simulink model "verify_Hot_Water_T_Mdot_Profile_mdl"  (R2018b)
settings: Solver=ode45  StartTime=0.0  StopTime=24*3600  MaxStep=900  RelTol=1e-3  EnableMultiTasking=on
undefined symbols (not defined in the file or in its folder): path_carnot
libraries: carnot x5
settings Model: DEBUGGLOBALLEVEL=DEBUGLEVEL  DEBUGMAXTOTALWARNINGS=0  DEBUGMAXCONSECUTIVEWARNINGS=0  DEBUGWRITETOFILE=0  DEBUGFILENAME='error.txt'  Creator=drhf  LastModifiedBy=P41573
settings DataIOCC: SaveFormat=Array  SignalLoggingSaveFormat=ModelDataLogs
settings OptimizationCC: ExpressionDepthLimit=2147483647  LifeSpan=inf
settings DebuggingCC: UnderspecifiedInitializationDetection=Classic  MergeDetectMultiDrivingBlocksExec=none  SolverPrmCheckMsg=warning  FcnCallInpInsideContextMsg=warning  StateNameClashWarn=warning  SFUnexpectedBacktrackingDiag=warning  SFNoUnconditionalDefaultTransitionDiag=warning  SFExecutionAtInitializationDiag=none
settings HardwareCC: ProdBitPerPointer=32  ProdBitPerSizeT=32  ProdBitPerPtrDiffT=32  ProdLargestAtomicFloat=None  ProdIntDivRoundTo=Undefined  ProdEndianess=Unspecified  ProdWordSize=32  ProdHWDeviceType=32-bit Generic
settings ModelReferenceCC: PropagateSignalLabelsOutOfModel=off
settings SFSimCC: SimUseLocalCustomCode=off
settings RTWCC: RTWUseLocalCustomCode=off
settings CodeAppCC: StateflowObjectComments=on
settings GRTTargetCC: TargetLangStandard=C89/C90 (ANSI)  GeneratePreprocessorConditionals=Disable all  CombineOutputUpdateFcns=off  GRTInterface=on
settings ConfigComp: CovMetricSettings=dw  CovHtmlReporting=on  CovSaveCumulativeToWorkspaceVar=on  CovSaveSingleToWorkspaceVar=on  CovExternalEMLEnable=off

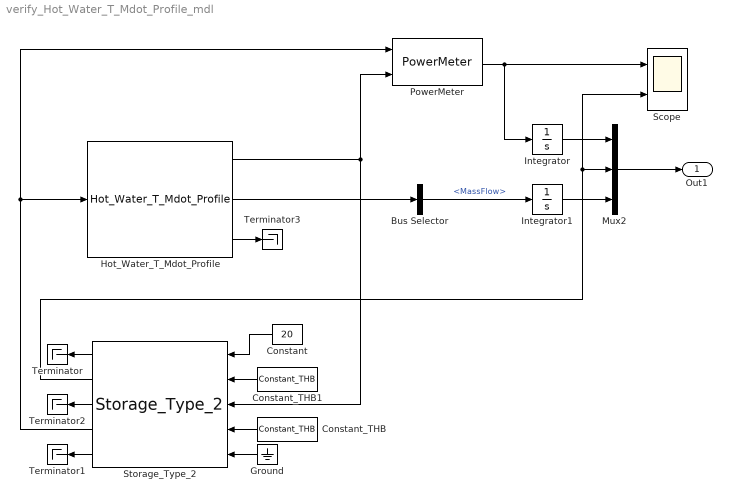
== system verify_Hot_Water_T_Mdot_Profile_mdl ==
  Bus Selector : BusSelector  OutputSignals=MassFlow
  Constant : Constant  Value=20
  Constant_THB : carnot/Source/Simple/Constant_THB  t=40  mdot=0*100/3600  p=1e5  mID=No Pressure Drop  fluid=Water  mix=0  mix2=0  mix3=0  dia=0.02  hgt=0
      settings: SourceProductName=Carnot
  Constant_THB1 : carnot/Source/Simple/Constant_THB  t=60  mdot=1000/3600  p=1e5  mID=No Pressure Drop  fluid=Water  mix=0  mix2=0  mix3=0  dia=0.02  hgt=0
      settings: SourceProductName=Carnot
  Ground : Ground
  Hot_Water_T_Mdot_Profile : carnot/Load/Hot_Water_Tapping/Hot_Water_T_Mdot_Profile  VariantControl=Variant3  Thot=45  Tcold=10  Tamp=0  dshift=-137  period="24*3600   % one day"  rep_seq_t="[7 12 19]*3600  % tapping at 7:00, 12:00 and 19:00"  rep_seq_d="[0.2 0.1 0.2]*3600  % total duration is 1/2 h"  rep_seq_y="[1 1 1]*200/1800   % 200 kg in 1/2 h"
      settings: SourceProductName=Carnot
  Integrator : Integrator
  Integrator1 : Integrator
  Mux2 : Mux  Inputs=3
  PowerMeter : carnot/Control/PowerMeter
      settings: SourceProductName=Carnot
  Scope : Scope  NumInputPorts=2
  Storage_Type_2 : carnot/Storage/Thermal/Storage_Type_2  t0=60  hgt=1.5279  stgtype=2  tini=[60 60 60 60 60 60 60 60 60 60]  mpts=[1 2 3 4 5 6 7 8 9 10]  PathName=fullfile(path_carnot('libsl'),'Storage','Thermal','Storage_Type_2','parameter_set')  FileName='StorageType2_300_L.mat'  userPath=off  userParam=off  uwall=1  ubot=1  utop=1  axcond=1  volume=0.3  dia=0.5  standing=standing cylinder  nodes=10  mpoints=10  Tsensor=0.5  hx1inlet=0.45  hx1outlet=0  hx1dia=0.03  hx1uac=50  hx1uam=0.15  hx1uat=0.6  uat2=0  hx1dpqua=20  hx1dplin=20  pipe1inlet=0  pipe1outlet=1  pipe1dia=0.03  pipe2inlet=0.6  pipe2outlet=1  pipe2dia=0.03  heater1start=0.6  heater1end=0.65
      settings: SourceProductName=Carnot
  Terminator{,1..3} (4 alike) : Terminator
  Out1 : Outport
  wires:
  Storage_Type_2/4 -> PowerMeter/1, Hot_Water_T_Mdot_Profile/1
  Hot_Water_T_Mdot_Profile/1 -> Storage_Type_2/3, PowerMeter/2
  Storage_Type_2/1 -> Terminator/1
  Constant_THB/1 -> Storage_Type_2/4
  Constant/1 -> Storage_Type_2/1
  Hot_Water_T_Mdot_Profile/3 -> Terminator3/1
  Hot_Water_T_Mdot_Profile/2 -> Bus Selector/1
  Mux2/1 -> Out1/1
  Storage_Type_2/2 -> Scope/2, Mux2/2
  Bus Selector/1 -> Integrator1/1  "<MassFlow>"
  PowerMeter/1 -> Integrator/1, Scope/1
  Integrator/1 -> Mux2/1
  Integrator1/1 -> Mux2/3
  Storage_Type_2/5 -> Terminator1/1
  Storage_Type_2/3 -> Terminator2/1
  Constant_THB1/1 -> Storage_Type_2/2
  Ground/1 -> Storage_Type_2/5
